simulink model "Problem6"  (R2020b)
settings: Solver=FixedStepAuto  StartTime=0.0  StopTime=10.0  RelTol=1e-3
settings Model: Creator=Administrator  LastModifiedBy=Administrator

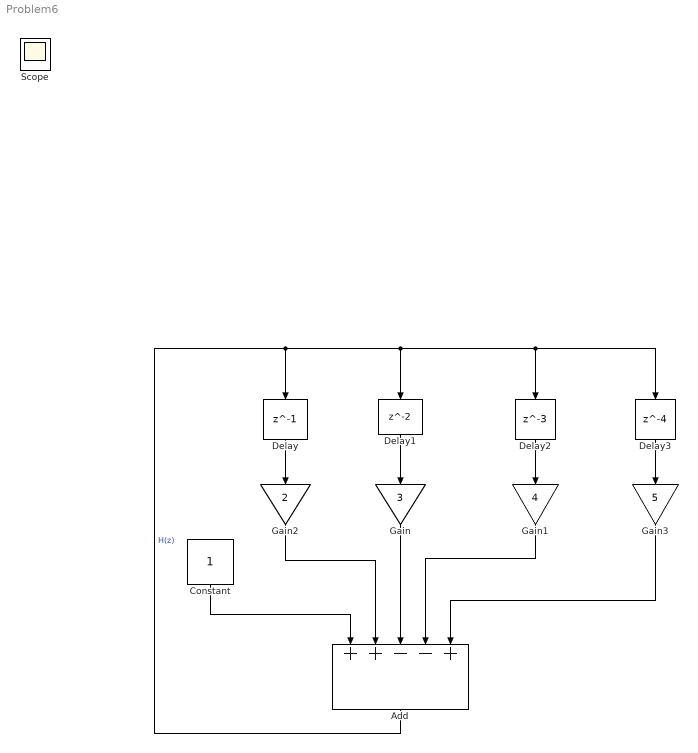
== system Problem6 ==
  Add : Sum  Inputs=++--+
  Constant : Constant
  Delay : Delay  DelayLength=1
  Delay1 : Delay
  Delay2 : Delay  DelayLength=3
  Delay3 : Delay  DelayLength=4
  Gain : Gain  Gain=3
  Gain1 : Gain  Gain=4
  Gain2 : Gain  Gain=2
  Gain3 : Gain  Gain=5
  Scope : Scope
  wires:
  Delay1/1 -> Gain/1
  Delay2/1 -> Gain1/1
  Delay3/1 -> Gain3/1
  Add/1 -> Delay3/1, Delay2/1, Delay1/1, Delay/1  "H(z)"
  Delay/1 -> Gain2/1
  Gain2/1 -> Add/2
  Gain/1 -> Add/3
  Gain1/1 -> Add/4
  Gain3/1 -> Add/5
  Constant/1 -> Add/1
